simulink model "CDMA2000sint_C_etapa6"
settings: Solver=ode45  StartTime=0.0  StopTime=200  RelTol=1e-3
libraries: commdigbbndpm3 x2, commrandsrc2 x1, commsink2 x1, simulink x1, commchan3 x1
settings Model: Creator=Oti  LastModifiedBy=Dan
settings DataIOCC: LimitDataPoints=on  SaveFormat=Array  SignalLoggingSaveFormat=ModelDataLogs  ReturnWorkspaceOutputs=off
settings OptimizationCC: ExpressionDepthLimit=2147483647  LifeSpan=inf  SimCompilerOptimization=Off
settings DebuggingCC: UnderspecifiedInitializationDetection=Classic  MergeDetectMultiDrivingBlocksExec=none  SolverPrmCheckMsg=warning  MultiTaskDSMMsg=warning  MultiTaskCondExecSysMsg=none  FcnCallInpInsideContextMsg=Enable All  FrameProcessingCompatibilityMsg=warning  StateNameClashWarn=warning  StrictBusMsg=None  SFUnexpectedBacktrackingDiag=warning  SFNoUnconditionalDefaultTransitionDiag=warning
settings HardwareCC: ProdBitPerPointer=32  ProdLargestAtomicFloat=None  ProdIntDivRoundTo=Undefined  ProdEndianess=Unspecified  ProdWordSize=32  ProdHWDeviceType=32-bit Generic
settings ModelReferenceCC: PropagateSignalLabelsOutOfModel=off
settings SFSimCC: SimUseLocalCustomCode=off
settings RTWCC: RTWUseLocalCustomCode=off  IncludeERTFirstTime=on  RTWCompilerOptimization=Off
settings CodeAppCC: CustomSymbolStrType=$N$R$M
settings GRTTargetCC: CodeReplacementLibrary=ANSI_C  GeneratePreprocessorConditionals=Disable all  CombineOutputUpdateFcns=off  CPPClassGenCompliant=off  GRTInterface=on

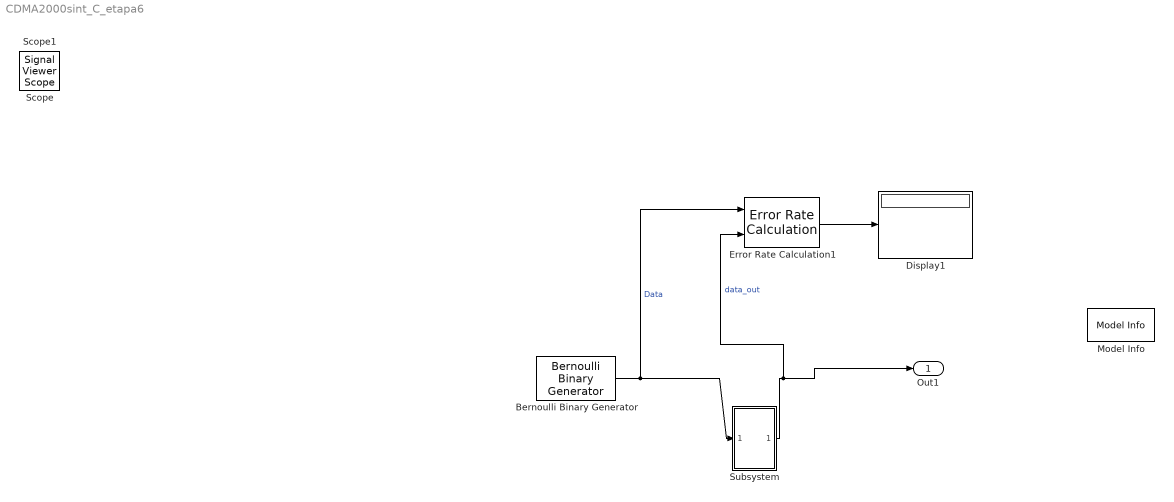
== system CDMA2000sint_C_etapa6 ==
  Bernoulli Binary Generator : commrandsrc2/Bernoulli Binary Generator  P=0.5  seed=61  Ts=1  frameBased=off  sampPerFrame=1  orient=off  outDataType=boolean
  Display1 : Display
  Error Rate Calculation1 : commsink2/Error Rate Calculation  N=0  st_delay=0  cp_mode=Entire frame  subframe=[]  PMode=Port  WsName=ErrorVec  RsMode2=off  stop=off  numErr=100  maxBits=1e6
  Model Info : simulink/Model-Wide Utilities/Model Info  InitialBlockCM=None  BlockCM=None  Frame=on  DisplayStringWithTags=SNR=6 dB  HorizontalTextAlignment=Left  LeftAlignmentValue=0.02  SourceBlockDiagram=CDMA2000sint_Craciun_etapa6  TagMaxNumber=20
  Subsystem : Subsystem
  Out1 : Outport
  Scope : SignalViewerScope  IOType=viewer  NumInputPorts=2  RefreshTime=0.035000
      settings: ShowDataMarkers=on  YMin=-5~-5  YMax=5~5
  Scope1 : SignalViewerScope  IOType=viewer  NumInputPorts=4  ZoomMode=xonly  RefreshTime=0.035000
      settings: TickLabels=on  ShowLegends=on  YMin=-5~-5~-5~-5  YMax=5~5~5~5
  wires:
  Subsystem/1(Out1) -> Error Rate Calculation1/2, Out1/1  "data_out"
  Error Rate Calculation1/1 -> Display1/1
  Bernoulli Binary Generator/1 -> Error Rate Calculation1/1, Subsystem/1(In1)  "Data"

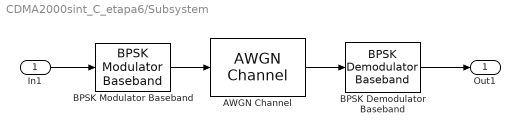
== system CDMA2000sint_C_etapa6/Subsystem ==
  In1 : Inport
  AWGN Channel : commchan3/AWGN Channel  InputProcessing=Columns as channels (frame based)  seed=67  noiseMode="Signal to noise ratio  (SNR)"  EbNodB=10  EsNodB=10  SNRdB=6  bitsPerSym=1  Ps=1  Tsym=1  variance=1
  BPSK Demodulator Baseband : commdigbbndpm3/BPSK Demodulator Baseband  Ph=0  DecType=Hard decision  VarSource=Dialog  Variance=1  outDtype=boolean  derotateFactorWordLen=16
  BPSK Modulator Baseband : commdigbbndpm3/BPSK Modulator Baseband  Ph=0  outDtype=double  outWordLen=16  outUDDataType=sfix(16)  outFracLenMode=Best precision  outFracLen=15
  Out1 : Outport
  wires:
  BPSK Modulator Baseband/1 -> AWGN Channel/1
  BPSK Demodulator Baseband/1 -> Out1/1
  AWGN Channel/1 -> BPSK Demodulator Baseband/1
  In1/1 -> BPSK Modulator Baseband/1
